simulink model "speed_loop"  (R2024b)
settings: Solver=VariableStepAuto  StartTime=0.0  StopTime=2  MaxStep=Ts/3  RelTol=1e-3
values from neighbouring files (symbols this model uses):
  Br = 1e-3    (= 0.001)    [IM_parameters_20250221.m]
  in = 3.2*sqrt(2)    [IM_parameters_20250221.m]
  Jcc = [0, -1; 1, 0]    [IM_parameters_20250221.m]
  Jr = 0.0055    [IM_parameters_20250221.m]
  Kiid = alpha_BW_i*(Rs+Rr)    (= 196524.073775)    [IM_parameters_20250221.m]
  Kiiq = alpha_BW_i*(Rs+Rr)    (= 196524.073775)    [IM_parameters_20250221.m]
  Kiw = Br*alpha_BW_w*sqrt(1+alpha_BW_w^2/alpha_BW_i^2)    [IM_parameters_20250221.m]
  Kpid = alpha_BW_i*Lsigma    (= 1012.29096616)    [IM_parameters_20250221.m]
  Kpiq = alpha_BW_i*Lsigma    (= 1012.29096616)    [IM_parameters_20250221.m]
  Kpw = Jr*alpha_BW_w*sqrt(1+alpha_BW_w^2/alpha_BW_i^2)    [IM_parameters_20250221.m]
  Lphi = 0.343    [IM_parameters_20250221.m]
  Lsigma = 0.029    [IM_parameters_20250221.m]
  p = 2    [IM_parameters_20250221.m]
  Rr = 2.66    [IM_parameters_20250221.m]
  Rs = 2.97    [IM_parameters_20250221.m]
  Ts = 10e-6    (= 1e-05)    [IM_parameters_20250221.m]
  un = 400    [IM_parameters_20250221.m]
libraries: simulink x1
settings Model: Creator=lucap  LastModifiedBy=guoxiaotao
settings RTWCC: GPUComputeCapability=3.5

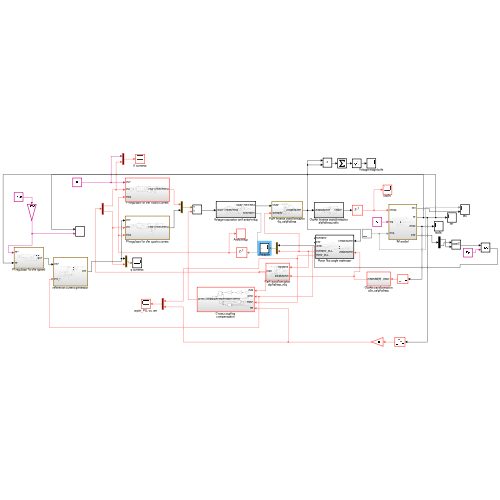
[thumbnail: Simulink's stored preview of the top-level diagram]
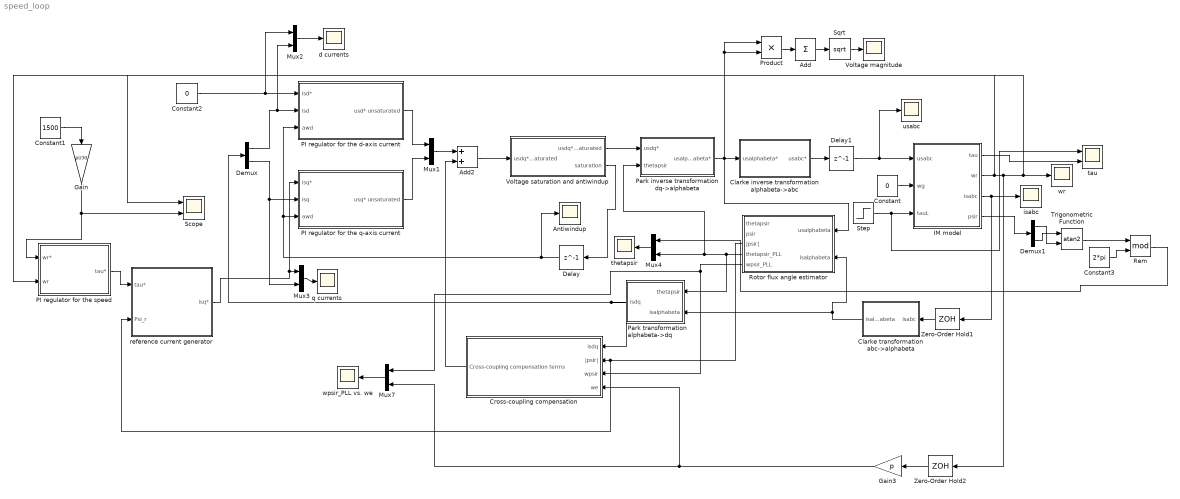
== system speed_loop ==
  Add : Sum  Inputs=+
  Add2 : Sum
  Antiwindup : Scope
  Clarke inverse transformation alphabeta->abc : Subsystem
  Clarke transformation abc->alphabeta : Subsystem
  Constant : Constant  Value=0
  Constant1 : Constant  Value=1500
  Constant2 : Constant  Value=0
  Constant3 : Constant  Value=2*pi
  Cross-coupling compensation : Subsystem
  Delay : Delay  DelayLength=1  SampleTime=Ts
  Delay1 : Delay  DelayLength=1  SampleTime=Ts
  Demux : Demux  Outputs=2
  Demux1 : Demux  Outputs=2
  Gain : Gain  Gain=pi/30
  Gain3 : Gain  Gain=p
  IM model : Subsystem
  Mux{1..4,7} (5 alike) : Mux  Inputs=2
  PI regulator for the d-axis current : Subsystem
  PI regulator for the q-axis current : Subsystem
  PI regulator for the speed : Subsystem
  Park inverse transformation dq->alphabeta : Subsystem
  Park transformation alphabeta->dq : Subsystem
  Product : Product
  Rem : Math  Operator=mod
  Rotor flux angle estimator : Subsystem
  Scope : Scope  NumInputPorts=2
  Sqrt : Sqrt
  Step : Step  Before=3  After=7  SampleTime=0
  Trigonometric Function : Trigonometry  Operator=atan2
  Voltage magnitude : Scope
  Voltage saturation and antiwindup : Subsystem
  Zero-Order Hold1 : ZeroOrderHold  SampleTime=Ts
  Zero-Order Hold2 : ZeroOrderHold  SampleTime=Ts
  d currents : Scope
  isabc : Scope
  q currents : Scope
  reference current generator : Subsystem
  tau : Scope  NumInputPorts=2
  thetapsir : Scope
  usabc : Scope
  wpsir_PLL vs. we : Scope
  wr : Scope
  wires:
  Mux2/1 -> d currents/1
  Sqrt/1 -> Voltage magnitude/1
  Mux1/1 -> Add2/1
  Mux3/1 -> q currents/1
  Zero-Order Hold1/1 -> Clarke transformation abc->alphabeta/1(isabc)
  Zero-Order Hold2/1 -> Gain3/1
  Add/1 -> Sqrt/1
  Clarke inverse transformation alphabeta->abc/1(usabc*) -> Delay1/1
  IM model/1(tau) -> tau/2
  Constant2/1 -> Mux2/1, PI regulator for the d-axis current/1(isd*)
  Delay1/1 -> IM model/1(usabc), usabc/1
  Gain3/1 -> Mux7/2, Cross-coupling compensation/4(we)
  IM model/3(isabc) -> Zero-Order Hold1/1, isabc/1
  PI regulator for the d-axis current/1(usd* unsaturated) -> Mux1/1
  Demux/1 -> Mux2/2, PI regulator for the d-axis current/2(isd)
  Product/1 -> Add/1
  Park transformation alphabeta->dq/1(isdq) -> Cross-coupling compensation/1(isdq), Demux/1
  Step/1 -> tau/1, IM model/3(tauL)
  Demux/2 -> Mux3/2, PI regulator for the q-axis current/2(isq)
  Delay/1 -> Antiwindup/1, PI regulator for the d-axis current/3(awd), PI regulator for the q-axis current/3(awd)
  PI regulator for the q-axis current/1(usq* unsaturated) -> Mux1/2
  Constant/1 -> IM model/2(wg)
  Clarke transformation abc->alphabeta/1(isalphabeta) -> Rotor flux angle estimator/2(isalphabeta), Park transformation alphabeta->dq/2(isalphabeta)
  Park inverse transformation dq->alphabeta/1(usalphabeta*) -> Rotor flux angle estimator/1(usalphabeta), Clarke inverse transformation alphabeta->abc/1(usalphabeta*), Product/2, Product/1
  IM model/4(psir) -> Demux1/1
  Trigonometric Function/1 -> Rem/1
  Constant3/1 -> Rem/2
  Demux1/2 -> Trigonometric Function/1
  Demux1/1 -> Trigonometric Function/2
  Mux4/1 -> thetapsir/1
  Rotor flux angle estimator/4(thetapsir_PLL) -> Park transformation alphabeta->dq/1(thetapsir), Park inverse transformation dq->alphabeta/2(thetapsir), Mux4/2
  Rotor flux angle estimator/5(wpsir_PLL) -> Cross-coupling compensation/3(wpsir), Mux7/1
  Mux7/1 -> wpsir_PLL vs. we/1
  Cross-coupling compensation/1(Cross-coupling compensation terms) -> Add2/2
  Rotor flux angle estimator/3(|psir|) -> reference current generator/2(Psi_r), Cross-coupling compensation/2(|psir|)
  Rem/1 -> Mux4/1
  Voltage saturation and antiwindup/2(saturation) -> Delay/1
  Voltage saturation and antiwindup/1(usdq* saturated) -> Park inverse transformation dq->alphabeta/1(usdq*)
  Add2/1 -> Voltage saturation and antiwindup/1(usdq* unsaturated)
  reference current generator/1(isq*) -> PI regulator for the q-axis current/1(isq*), Mux3/1
  PI regulator for the speed/1(tau*) -> reference current generator/1(tau*)
  Constant1/1 -> Gain/1
  IM model/2(wr) -> PI regulator for the speed/2(wr), Zero-Order Hold2/1, Scope/1, wr/1
  Gain/1 -> PI regulator for the speed/1(wr*), Scope/2

== system speed_loop/Clarke inverse transformation alphabeta->abc ==
  usalphabeta* : Inport
  Add5 : Sum  Inputs=-+
  Add6 : Sum  Inputs=--
  Demux : Demux  Outputs=2
  Gain6 : Gain  Gain=0.5
  Gain7 : Gain  Gain=sqrt(3)
  Gain8 : Gain  Gain=0.5
  Mux : Mux  Inputs=3
  usabc* : Outport
  wires:
  Demux/1 -> Mux/1, Add6/1, Add5/1
  Demux/2 -> Gain7/1
  Add5/1 -> Gain6/1
  Gain7/1 -> Add6/2, Add5/2
  Gain6/1 -> Mux/2
  Add6/1 -> Gain8/1
  Gain8/1 -> Mux/3
  usalphabeta*/1 -> Demux/1
  Mux/1 -> usabc*/1

== system speed_loop/Clarke transformation abc->alphabeta ==
  isabc : Inport
  Add : Sum  Inputs=+--
  Add1 : Sum  Inputs=+-
  Add2 : Sum
  Constant : Constant  Value=[0 0 0]
  Demux : Demux  Outputs=3
  Gain : Gain  Gain=2
  Gain3 : Gain  Gain=sqrt(3)/3
  Gain4 : Gain  Gain=1/3
  Mux : Mux  Inputs=2
  isalphabeta : Outport
  wires:
  Add1/1 -> Gain3/1
  Add/1 -> Gain4/1
  Gain/1 -> Add/1
  Demux/2 -> Add1/1, Add/2
  Demux/3 -> Add1/2, Add/3
  isabc/1 -> Add2/1
  Demux/1 -> Gain/1
  Mux/1 -> isalphabeta/1
  Gain4/1 -> Mux/1
  Gain3/1 -> Mux/2
  Add2/1 -> Demux/1
  Constant/1 -> Add2/2

== system speed_loop/Cross-coupling compensation ==
  isdq : Inport
  |psir| : Inport  Port=2
  wpsir : Inport  Port=3
  we : Inport  Port=4
  Add : Sum
  Gain : Gain  Gain=Lsigma
  Gain1 : Gain  Gain=-Rr/Lphi
  Gain2 : Gain  Gain=Jcc  Multiplication=Matrix(K*u)
  Mux : Mux  Inputs=2
  Product : Product
  Product1 : Product
  Cross-coupling compensation terms : Outport
  wires:
  Add/1 -> Cross-coupling compensation terms/1
  isdq/1 -> Gain2/1
  Gain2/1 -> Gain/1
  Gain/1 -> Product/1
  wpsir/1 -> Product/2
  Product1/1 -> Mux/2
  Gain1/1 -> Mux/1
  Product/1 -> Add/1
  Mux/1 -> Add/2
  |psir|/1 -> Product1/1, Gain1/1
  we/1 -> Product1/2

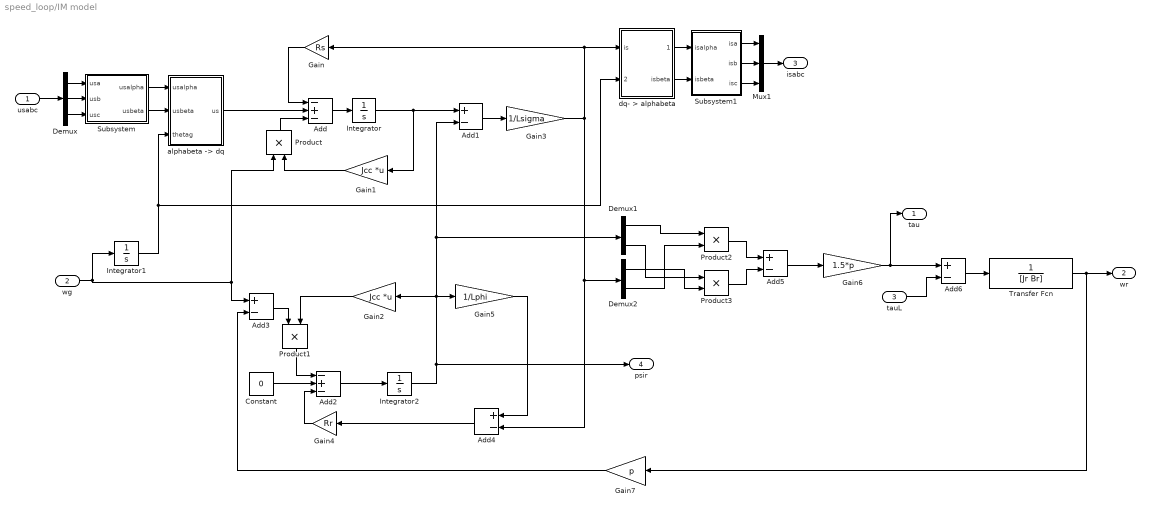
== system speed_loop/IM model ==
  usabc : Inport
  wg : Inport  Port=2
  tauL : Inport  Port=3
  Add : Sum  Inputs=-+-
  Add{1,3..6} (5 alike) : Sum  Inputs=+-
  Add2 : Sum  Inputs=-+-
  Constant : Constant  Value=0
  Demux : Demux  Outputs=3
  Demux1 : Demux  Outputs=2
  Demux2 : Demux  Outputs=2
  Gain : Gain  Gain=Rs
  Gain1 : Gain  Gain=Jcc  Multiplication=Matrix(K*u)
  Gain2 : Gain  Gain=Jcc  Multiplication=Matrix(K*u)
  Gain3 : Gain  Gain=1/Lsigma
  Gain4 : Gain  Gain=Rr
  Gain5 : Gain  Gain=1/Lphi
  Gain6 : Gain  Gain=1.5*p
  Gain7 : Gain  Gain=p
  Integrator : Integrator
  Integrator1 : Integrator
  Integrator2 : Integrator
  Mux1 : Mux  Inputs=3
  Product{,1..3} (4 alike) : Product
  Subsystem : Subsystem
  Subsystem1 : Subsystem
  Transfer Fcn : TransferFcn  Denominator=[Jr Br]
  "alphabeta -> dq" : Subsystem
  dq- > alphabeta : Subsystem
  tau : Outport
  wr : Outport  Port=2
  isabc : Outport  Port=3
  psir : Outport  Port=4
  wires:
  Subsystem/2(usbeta) -> "alphabeta -> dq"/2(usbeta)
  Subsystem/1(usalpha) -> "alphabeta -> dq"/1(usalpha)
  dq- > alphabeta/1(isalpha) -> Subsystem1/1(isalpha)
  dq- > alphabeta/2(isbeta) -> Subsystem1/2(isbeta)
  Mux1/1 -> isabc/1
  Subsystem1/2(isb) -> Mux1/2
  Subsystem1/1(isa) -> Mux1/1
  Subsystem1/3(isc) -> Mux1/3
  usabc/1 -> Demux/1
  Demux/1 -> Subsystem/1(usa)
  Demux/2 -> Subsystem/2(usb)
  Demux/3 -> Subsystem/3(usc)
  Gain/1 -> Add/1
  Add/1 -> Integrator/1
  Integrator/1 -> Add1/1, Gain1/1
  wg/1 -> Add3/1, Product/1, Integrator1/1
  Integrator1/1 -> dq- > alphabeta/2(thetag), "alphabeta -> dq"/3(thetag)
  Product/1 -> Add/3
  Gain1/1 -> Product/2
  "alphabeta -> dq"/1(us) -> Add/2
  Add1/1 -> Gain3/1
  Gain3/1 -> Demux2/1, Add4/2, dq- > alphabeta/1(is), Gain/1
  Constant/1 -> Add2/2
  Gain4/1 -> Add2/3
  Product1/1 -> Add2/1
  Add2/1 -> Integrator2/1
  Gain7/1 -> Add3/2
  Add3/1 -> Product1/1
  Gain2/1 -> Product1/2
  Add4/1 -> Gain4/1
  Integrator2/1 -> psir/1, Gain2/1, Gain5/1, Demux1/1, Add1/2
  Gain5/1 -> Add4/1
  Add5/1 -> Gain6/1
  Product2/1 -> Add5/1
  Product3/1 -> Add5/2
  Demux1/1 -> Product2/1
  Demux2/2 -> Product2/2
  Demux1/2 -> Product3/1
  Demux2/1 -> Product3/2
  tauL/1 -> Add6/2
  Gain6/1 -> tau/1, Add6/1
  Add6/1 -> Transfer Fcn/1
  Transfer Fcn/1 -> wr/1, Gain7/1

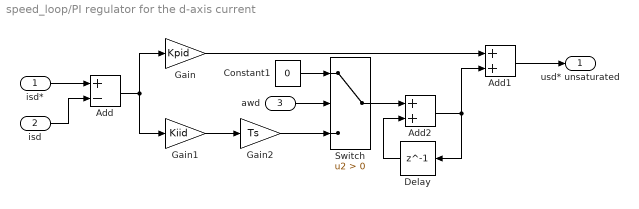
== system speed_loop/PI regulator for the d-axis current ==
  isd* : Inport
  isd : Inport  Port=2
  awd : Inport  Port=3
  Add : Sum  Inputs=+-
  Add1 : Sum
  Add2 : Sum
  Constant1 : Constant  Value=0
  Delay : Delay  DelayLength=1  SampleTime=Ts
  Gain : Gain  Gain=Kpid
  Gain1 : Gain  Gain=Kiid
  Gain2 : Gain  Gain=Ts
  Switch : Switch  Criteria=u2 > Threshold  SaturateOnIntegerOverflow=off  InputSameDT=off
  usd* unsaturated : Outport
  wires:
  Constant1/1 -> Switch/1
  Switch/1 -> Add2/1
  isd*/1 -> Add/1
  Add2/1 -> Delay/1, Add1/2
  isd/1 -> Add/2
  Add/1 -> Gain1/1, Gain/1
  Delay/1 -> Add2/2
  Gain1/1 -> Gain2/1
  Gain/1 -> Add1/1
  awd/1 -> Switch/2
  Add1/1 -> usd* unsaturated/1
  Gain2/1 -> Switch/3

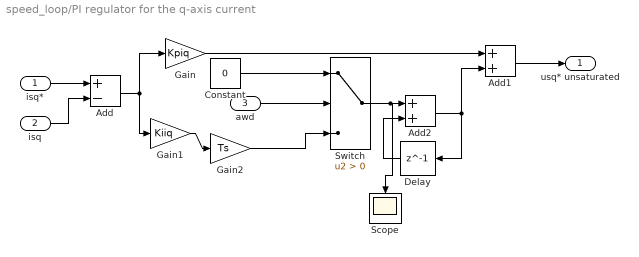
== system speed_loop/PI regulator for the q-axis current ==
  isq* : Inport
  isq : Inport  Port=2
  awd : Inport  Port=3
  Add : Sum  Inputs=+-
  Add1 : Sum
  Add2 : Sum
  Constant : Constant  Value=0
  Delay : Delay  DelayLength=1  SampleTime=Ts
  Gain : Gain  Gain=Kpiq
  Gain1 : Gain  Gain=Kiiq
  Gain2 : Gain  Gain=Ts
  Scope : Scope
  Switch : Switch  Criteria=u2 > Threshold  SaturateOnIntegerOverflow=off  InputSameDT=off
  usq* unsaturated : Outport
  wires:
  Add1/1 -> usq* unsaturated/1
  awd/1 -> Switch/2
  Gain/1 -> Add1/1
  Gain1/1 -> Gain2/1
  Delay/1 -> Add2/2
  Add/1 -> Gain/1, Gain1/1
  isq/1 -> Add/2
  Add2/1 -> Add1/2, Delay/1
  isq*/1 -> Add/1
  Switch/1 -> Scope/1, Add2/1
  Gain2/1 -> Switch/3
  Constant/1 -> Switch/1

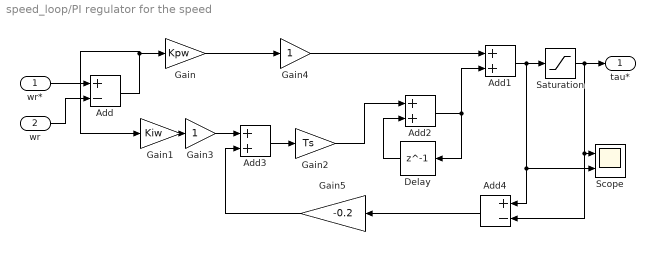
== system speed_loop/PI regulator for the speed ==
  wr* : Inport
  wr : Inport  Port=2
  Add : Sum  Inputs=+-
  Add1 : Sum
  Add2 : Sum
  Add3 : Sum
  Add4 : Sum  Inputs=+-
  Delay : Delay  DelayLength=1  SampleTime=Ts
  Gain : Gain  Gain=Kpw
  Gain1 : Gain  Gain=Kiw
  Gain2 : Gain  Gain=Ts
  Gain3 : Gain
  Gain4 : Gain
  Gain5 : Gain  Gain=-0.2
  Saturation : Saturate  UpperLimit=10  LowerLimit=-10
  Scope : Scope  NumInputPorts=2
  tau* : Outport
  wires:
  Delay/1 -> Add2/2
  Add/1 -> Gain/1, Gain1/1
  Add2/1 -> Add1/2, Delay/1
  Add1/1 -> Scope/2, Add4/1, Saturation/1
  Gain2/1 -> Add2/1
  Add3/1 -> Gain2/1
  Saturation/1 -> Scope/1, Add4/2, tau*/1
  Add4/1 -> Gain5/1
  Gain/1 -> Gain4/1
  Gain1/1 -> Gain3/1
  Gain3/1 -> Add3/1
  Gain4/1 -> Add1/1
  wr*/1 -> Add/1
  wr/1 -> Add/2
  Gain5/1 -> Add3/2

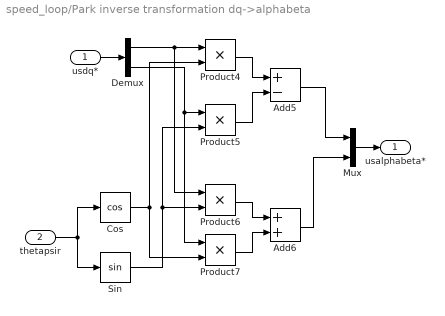
== system speed_loop/Park inverse transformation dq->alphabeta ==
  usdq* : Inport
  thetapsir : Inport  Port=2
  Add5 : Sum  Inputs=+-
  Add6 : Sum
  Cos : Trigonometry  Operator=cos
  Demux : Demux  Outputs=2
  Mux : Mux  Inputs=2
  Product{4..7} (4 alike) : Product
  Sin : Trigonometry
  usalphabeta* : Outport
  wires:
  Add6/1 -> Mux/2
  Add5/1 -> Mux/1
  thetapsir/1 -> Cos/1, Sin/1
  Demux/1 -> Product6/1, Product4/1
  Product7/1 -> Add6/2
  Product5/1 -> Add5/2
  Cos/1 -> Product4/2, Product7/2
  Sin/1 -> Product5/2, Product6/2
  Product4/1 -> Add5/1
  Demux/2 -> Product5/1, Product7/1
  Product6/1 -> Add6/1
  usdq*/1 -> Demux/1
  Mux/1 -> usalphabeta*/1

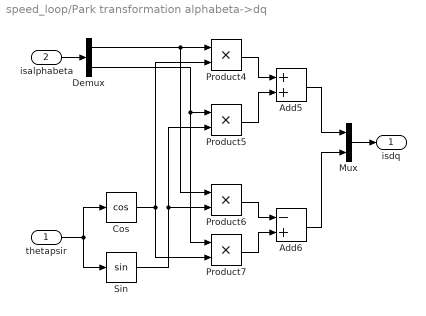
== system speed_loop/Park transformation alphabeta->dq ==
  thetapsir : Inport
  isalphabeta : Inport  Port=2
  Add5 : Sum
  Add6 : Sum  Inputs=-+
  Cos : Trigonometry  Operator=cos
  Demux : Demux  Outputs=2
  Mux : Mux  Inputs=2
  Product{4..7} (4 alike) : Product
  Sin : Trigonometry
  isdq : Outport
  wires:
  Product6/1 -> Add6/1
  Demux/2 -> Product7/1, Product5/1
  Product4/1 -> Add5/1
  Sin/1 -> Product6/2, Product5/2
  Cos/1 -> Product7/2, Product4/2
  Product5/1 -> Add5/2
  Product7/1 -> Add6/2
  Demux/1 -> Product6/1, Product4/1
  thetapsir/1 -> Sin/1, Cos/1
  Add6/1 -> Mux/2
  isalphabeta/1 -> Demux/1
  Add5/1 -> Mux/1
  Mux/1 -> isdq/1

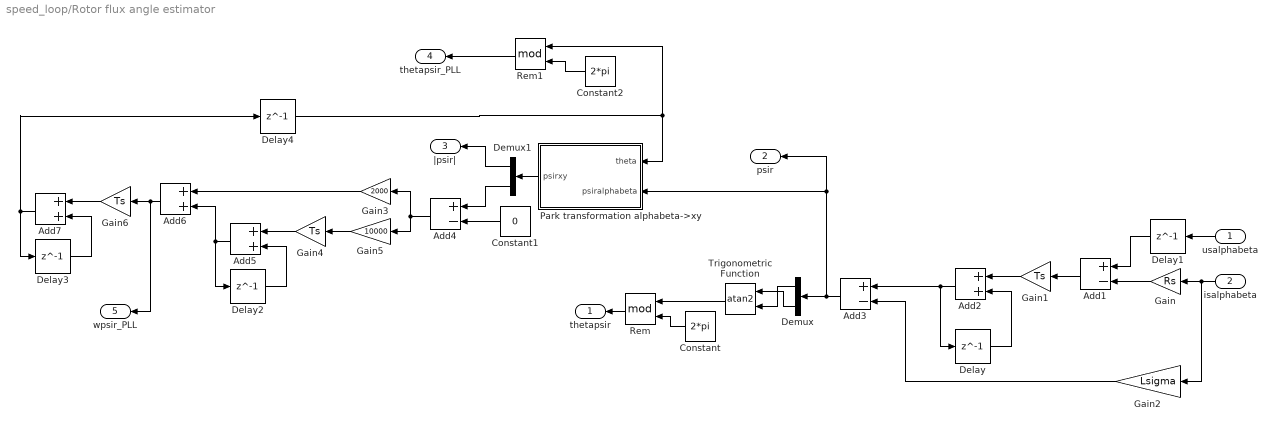
== system speed_loop/Rotor flux angle estimator ==
  usalphabeta : Inport
  isalphabeta : Inport  Port=2
  Add1 : Sum  Inputs=+-
  Add{2,5..7} (4 alike) : Sum
  Add3 : Sum  Inputs=+-
  Add4 : Sum  Inputs=+-
  Constant : Constant  Value=2*pi
  Constant1 : Constant  Value=0
  Constant2 : Constant  Value=2*pi
  Delay{,1..4} (5 alike) : Delay  DelayLength=1  SampleTime=Ts
  Demux : Demux  Outputs=2
  Demux1 : Demux  Outputs=2
  Gain : Gain  Gain=Rs
  Gain1 : Gain  Gain=Ts
  Gain2 : Gain  Gain=Lsigma
  Gain3 : Gain  Gain=2000
  Gain4 : Gain  Gain=Ts
  Gain5 : Gain  Gain=10000
  Gain6 : Gain  Gain=Ts
  Park transformation alphabeta->xy : Subsystem
  Rem : Math  Operator=mod
  Rem1 : Math  Operator=mod
  Trigonometric Function : Trigonometry  Operator=atan2
  thetapsir : Outport
  psir : Outport  Port=2
  |psir| : Outport  Port=3
  thetapsir_PLL : Outport  Port=4
  wpsir_PLL : Outport  Port=5
  wires:
  Gain/1 -> Add1/2
  isalphabeta/1 -> Gain/1, Gain2/1
  Delay/1 -> Add2/2
  Add1/1 -> Gain1/1
  Gain1/1 -> Add2/1
  Add2/1 -> Add3/1, Delay/1
  Gain2/1 -> Add3/2
  Add3/1 -> psir/1, Park transformation alphabeta->xy/2(psiralphabeta), Demux/1
  Trigonometric Function/1 -> Rem/1
  Demux/2 -> Trigonometric Function/1
  Demux/1 -> Trigonometric Function/2
  usalphabeta/1 -> Delay1/1
  Constant/1 -> Rem/2
  Rem/1 -> thetapsir/1
  Delay1/1 -> Add1/1
  Park transformation alphabeta->xy/1(psirxy) -> Demux1/1
  Demux1/1 -> |psir|/1
  Demux1/2 -> Add4/1
  Constant1/1 -> Add4/2
  Add5/1 -> Add6/2, Delay2/1
  Gain4/1 -> Add5/1
  Delay2/1 -> Add5/2
  Gain5/1 -> Gain4/1
  Add4/1 -> Gain5/1, Gain3/1
  Gain3/1 -> Add6/1
  Delay3/1 -> Add7/2
  Gain6/1 -> Add7/1
  Add6/1 -> wpsir_PLL/1, Gain6/1
  Add7/1 -> Delay4/1, Delay3/1
  Constant2/1 -> Rem1/2
  Delay4/1 -> Rem1/1, Park transformation alphabeta->xy/1(theta)
  Rem1/1 -> thetapsir_PLL/1

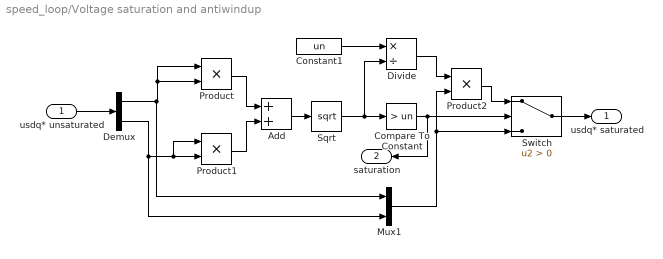
== system speed_loop/Voltage saturation and antiwindup ==
  usdq* unsaturated : Inport
  Add : Sum
  Compare To Constant : simulink/Logic and Bit Operations/Compare To Constant  relop=>  const=un  OutDataTypeStr=boolean
  Constant1 : Constant  Value=un
  Demux : Demux  Outputs=2
  Divide : Product  Inputs=*/
  Mux1 : Mux  Inputs=2
  Product : Product
  Product1 : Product
  Product2 : Product
  Sqrt : Sqrt
  Switch : Switch  Criteria=u2 > Threshold  SaturateOnIntegerOverflow=off  InputSameDT=off
  usdq* saturated : Outport
  saturation : Outport  Port=2
  wires:
  Constant1/1 -> Divide/1
  Switch/1 -> usdq* saturated/1
  Divide/1 -> Product2/1
  Product1/1 -> Add/2
  Mux1/1 -> Switch/3, Product2/2
  Demux/2 -> Product1/2, Product1/1, Mux1/2
  Demux/1 -> Mux1/1, Product/1, Product/2
  Compare To Constant/1 -> saturation/1, Switch/2
  Add/1 -> Sqrt/1
  Product/1 -> Add/1
  Product2/1 -> Switch/1
  usdq* unsaturated/1 -> Demux/1
  Sqrt/1 -> Divide/2, Compare To Constant/1

== system speed_loop/reference current generator ==
  tau* : Inport
  Psi_r : Inport  Port=2
  Add : Sum
  Divide : Product  Inputs=*/
  Gain : Gain  Gain=1.5
  Gain1 : Gain  Gain=p
  Saturation : Saturate  UpperLimit=in*10  LowerLimit=-in*5
  Scope : Scope  NumInputPorts=2
  Scope1 : Scope
  Step : Step  Time=0.1  Before=0.1  After=0  SampleTime=0
  isq* : Outport
  wires:
  tau*/1 -> Divide/1
  Gain/1 -> Gain1/1
  Psi_r/1 -> Gain/1
  Gain1/1 -> Scope1/1, Add/2
  Add/1 -> Divide/2
  Saturation/1 -> Scope/2, isq*/1
  Step/1 -> Add/1
  Divide/1 -> Scope/1, Saturation/1

== system speed_loop/IM model/Subsystem ==
  usa : Inport
  usb : Inport  Port=2
  usc : Inport  Port=3
  Add5 : Sum  Inputs=+--
  Add6 : Sum  Inputs=+-
  Gain10 : Gain  Gain=sqrt(3)/3
  Gain11 : Gain  Gain=sqrt(3)/3
  Gain7 : Gain  Gain=0.5
  Gain8 : Gain  Gain=0.5
  Gain9 : Gain  Gain=2/3
  usalpha : Outport
  usbeta : Outport  Port=2
  wires:
  Gain11/1 -> Add6/2
  usc/1 -> Gain11/1, Gain8/1
  Add5/1 -> Gain9/1
  Gain10/1 -> Add6/1
  usb/1 -> Gain10/1, Gain7/1
  usa/1 -> Add5/1
  Add6/1 -> usbeta/1
  Gain8/1 -> Add5/3
  Gain7/1 -> Add5/2
  Gain9/1 -> usalpha/1

== system speed_loop/IM model/Subsystem1 ==
  isalpha : Inport
  isbeta : Inport  Port=2
  Add5 : Sum  Inputs=-+
  Add6 : Sum  Inputs=--
  Gain1 : Gain  Gain=0.5
  Gain2 : Gain  Gain=0.5
  Gain8 : Gain  Gain=sqrt(3)
  isa : Outport
  isb : Outport  Port=2
  isc : Outport  Port=3
  wires:
  isbeta/1 -> Gain8/1
  isalpha/1 -> Add6/1, Add5/1, isa/1
  Gain8/1 -> Add6/2, Add5/2
  Add5/1 -> Gain1/1
  Gain1/1 -> isb/1
  Add6/1 -> Gain2/1
  Gain2/1 -> isc/1

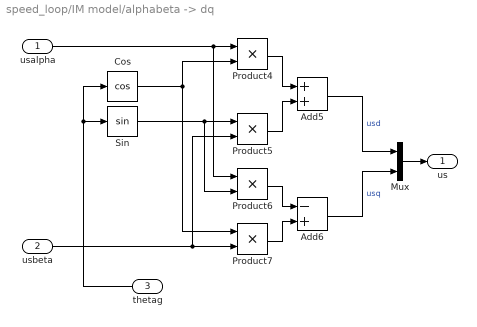
== system speed_loop/IM model/alphabeta -> dq ==
  usalpha : Inport
  usbeta : Inport  Port=2
  thetag : Inport  Port=3
  Add5 : Sum
  Add6 : Sum  Inputs=-+
  Cos : Trigonometry  Operator=cos
  Mux : Mux  Inputs=2
  Product{4..7} (4 alike) : Product
  Sin : Trigonometry
  us : Outport
  wires:
  Product4/1 -> Add5/1
  Sin/1 -> Product6/2, Product5/1
  usbeta/1 -> Product5/2, Product7/2
  Product6/1 -> Add6/1
  Cos/1 -> Product7/1, Product4/2
  usalpha/1 -> Product6/1, Product4/1
  Product5/1 -> Add5/2
  Product7/1 -> Add6/2
  thetag/1 -> Sin/1, Cos/1
  Add5/1 -> Mux/1  "usd"
  Add6/1 -> Mux/2  "usq"
  Mux/1 -> us/1

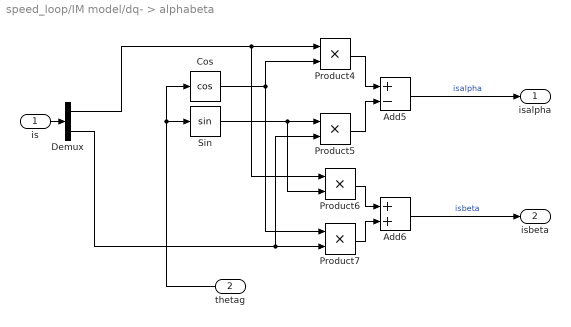
== system speed_loop/IM model/dq- > alphabeta ==
  is : Inport
  thetag : Inport  Port=2
  Add5 : Sum  Inputs=+-
  Add6 : Sum
  Cos : Trigonometry  Operator=cos
  Demux : Demux  Outputs=2
  Product{4..7} (4 alike) : Product
  Sin : Trigonometry
  isalpha : Outport
  isbeta : Outport  Port=2
  wires:
  thetag/1 -> Cos/1, Sin/1
  Product7/1 -> Add6/2
  Product5/1 -> Add5/2
  Cos/1 -> Product4/2, Product7/1
  Product6/1 -> Add6/1
  Demux/2 -> Product7/2, Product5/2
  Sin/1 -> Product5/1, Product6/2
  Product4/1 -> Add5/1
  Add5/1 -> isalpha/1  "isalpha"
  Add6/1 -> isbeta/1  "isbeta"
  Demux/1 -> Product6/1, Product4/1
  is/1 -> Demux/1

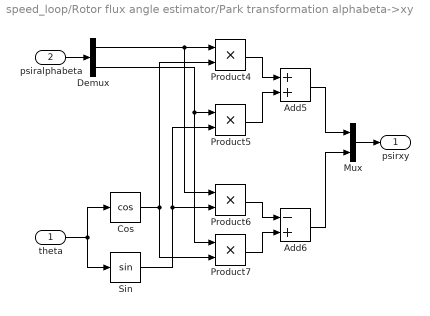
== system speed_loop/Rotor flux angle estimator/Park transformation alphabeta->xy ==
  theta : Inport
  psiralphabeta : Inport  Port=2
  Add5 : Sum
  Add6 : Sum  Inputs=-+
  Cos : Trigonometry  Operator=cos
  Demux : Demux  Outputs=2
  Mux : Mux  Inputs=2
  Product{4..7} (4 alike) : Product
  Sin : Trigonometry
  psirxy : Outport
  wires:
  Mux/1 -> psirxy/1
  Add5/1 -> Mux/1
  psiralphabeta/1 -> Demux/1
  Add6/1 -> Mux/2
  theta/1 -> Cos/1, Sin/1
  Demux/1 -> Product4/1, Product6/1
  Product7/1 -> Add6/2
  Product5/1 -> Add5/2
  Cos/1 -> Product4/2, Product7/2
  Sin/1 -> Product5/2, Product6/2
  Product4/1 -> Add5/1
  Demux/2 -> Product5/1, Product7/1
  Product6/1 -> Add6/1
